simulink model "Misil_Simulinknobus"  (R2021b)
settings: Solver=VariableStepAuto  StartTime=0.0  StopTime=10  FixedStep=0.001  RelTol=1e-3  EnableMultiTasking=on
PreLoadFcn:
  | codigos
libraries: aerolibanim x1, aerolibatmos2 x1
settings Model: Creator=usuario  LastModifiedBy=verti
settings SolverCC: AlgebraicLoopSolver=TrustRegion
settings DataIOCC: LimitDataPoints=on  SaveFormat=Array  SignalLoggingSaveFormat=ModelDataLogs  ReturnWorkspaceOutputs=off
settings OptimizationCC: ExpressionDepthLimit=2147483647  LifeSpan=inf
settings DebuggingCC: UnderspecifiedInitializationDetection=Classic  MergeDetectMultiDrivingBlocksExec=none  SolverPrmCheckMsg=warning  FcnCallInpInsideContextMsg=warning  StateNameClashWarn=warning  SFUnexpectedBacktrackingDiag=warning  SFNoUnconditionalDefaultTransitionDiag=warning  SFExecutionAtInitializationDiag=none  SFMachineParentedDataDiag=warning  ArithmeticOperatorsInVariantConditions=warning
settings HardwareCC: ProdBitPerPointer=32  ProdBitPerSizeT=32  ProdBitPerPtrDiffT=32  ProdLargestAtomicFloat=None  ProdIntDivRoundTo=Undefined  ProdEndianess=Unspecified  ProdWordSize=32  ProdHWDeviceType=32-bit Generic
settings ModelReferenceCC: PropagateSignalLabelsOutOfModel=off
settings SFSimCC: SimUseLocalCustomCode=off  CustomCodeUndefinedFunction=UseInterfaceOnly
settings RTWCC: RTWUseLocalCustomCode=off
settings CodeAppCC: StateflowObjectComments=on
settings GRTTargetCC: TargetLangStandard=C89/C90 (ANSI)  CombineOutputUpdateFcns=off  GRTInterface=on
settings ConfigComp: CovMetricSettings=dw  CovSaveCumulativeToWorkspaceVar=on  CovSaveSingleToWorkspaceVar=on  CovExternalEMLEnable=off

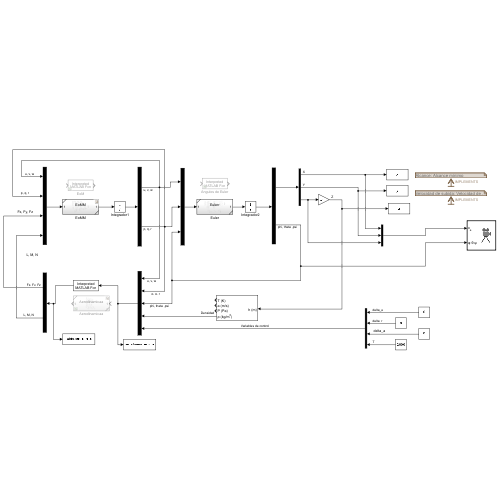
[thumbnail: Simulink's stored preview of the top-level diagram]
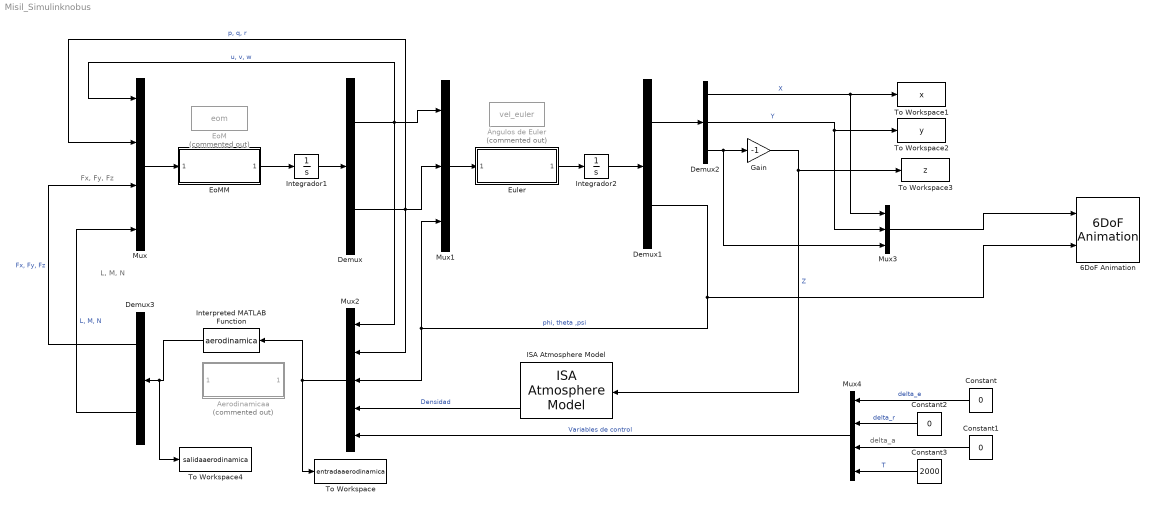
== system Misil_Simulinknobus ==
  note: delta_a
  note: Fx, Fy, Fz
  note: L, M, N
  6DoF Animation : aerolibanim/6DoF Animation  u1=[0 4000 0 4000 0 4000]  u2=0.1  u3=20  u4=[0 0 0]  u5=Fly alongside  u6=[200 200 200]  u7=10  u8=on
  Aerodinamicaa : Subsystem  Commented=on  ReferencedSubsystem=Aerodinamicaa
  Constant : Constant  Value=0
  Constant1 : Constant  Value=0
  Constant2 : Constant  Value=0
  Constant3 : Constant  Value=2000
  Demux : Demux  Outputs=2
  Demux1 : Demux  Outputs=2
  Demux2 : Demux  Outputs=3
  Demux3 : Demux  Outputs=2
  EoM : MATLABFcn  Commented=on  MATLABFcn=eom  OutputDimensions=6
  EoMM : Subsystem  ReferencedSubsystem=EoMM
  Euler : Subsystem  ReferencedSubsystem=Eulerr
  Gain : Gain  Gain=-1
  ISA Atmosphere Model : aerolibatmos2/ISA Atmosphere Model  custom=off  g=9.80665  gamma=1.4  R=287.0531  L=0.0065  h_trop=11000  h_strat=20000  rho0=1.225  P0=101325  T0=288.15  h0=0
  Integrador1 : Integrator  InitialCondition=[0.001,0,0,0,0,0]
  Integrador2 : Integrator  InitialCondition=[0,0,2000,0,pi/4,0]
      settings: DeleteFcn=slcm Cancel;  NameChangeFcn=slcm Rename;
  Interpreted MATLAB Function : MATLABFcn  MATLABFcn=aerodinamica  OutputDimensions=6
  Mux : Mux
  Mux1 : Mux  Inputs=3
  Mux2 : Mux  Inputs=5
  Mux3 : Mux  Inputs=3
  Mux4 : Mux
  To Workspace : ToWorkspace  VariableName=entradaaerodinamica  SaveFormat=Structure With Time  SampleTime=-1
  To Workspace1 : ToWorkspace  VariableName=x  SampleTime=-1
  To Workspace2 : ToWorkspace  VariableName=y  SampleTime=-1
  To Workspace3 : ToWorkspace  VariableName=z  SampleTime=-1
  To Workspace4 : ToWorkspace  VariableName=salidaaerodinamica  SaveFormat=Structure With Time  SampleTime=-1
  Ángulos de Euler : MATLABFcn  Commented=on  MATLABFcn=vel_euler  OutputDimensions=6
  wires:
  Integrador1/1 -> Demux/1
  Mux1/1 -> Euler/1
  Integrador2/1 -> Demux1/1
  Demux1/1 -> Demux2/1
  Demux/2 -> Mux2/2, Mux/2, Mux1/2  "p, q, r"
  Demux1/2 -> 6DoF Animation/2, Mux2/3, Mux1/3  "phi, theta ,psi"
  Demux2/3 -> Gain/1, Mux3/3
  Gain/1 -> ISA Atmosphere Model/1, To Workspace3/1  "Z"
  Demux2/1 -> Mux3/1, To Workspace1/1  "X"
  Demux2/2 -> Mux3/2, To Workspace2/1  "Y"
  Constant3/1 -> Mux4/4  "T"
  Constant1/1 -> Mux4/3
  Constant2/1 -> Mux4/2  "delta_r"
  Constant/1 -> Mux4/1  "delta_e"
  Demux3/1 -> Mux/3  "Fx, Fy, Fz"
  Demux3/2 -> Mux/4  "L, M, N"
  ISA Atmosphere Model/4 -> Mux2/4  "Densidad"
  Mux4/1 -> Mux2/5  "Variables de control"
  Mux3/1 -> 6DoF Animation/1
  Demux/1 -> Mux2/1, Mux/1, Mux1/1  "u, v, w"
  Mux2/1 -> Interpreted MATLAB Function/1, To Workspace/1
  Mux/1 -> EoMM/1
  EoMM/1 -> Integrador1/1
  Euler/1 -> Integrador2/1
  Interpreted MATLAB Function/1 -> To Workspace4/1, Demux3/1
